simulink model "simulink"  (R2023a)
settings: Solver=VariableStepAuto  StartTime=0.0  StopTime=10.0  RelTol=1e-3
settings Model: Creator=chirag  LastModifiedBy=chirag

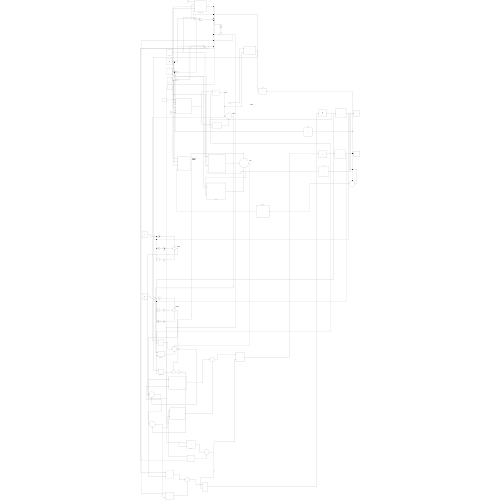
[thumbnail: Simulink's stored preview of the top-level diagram]
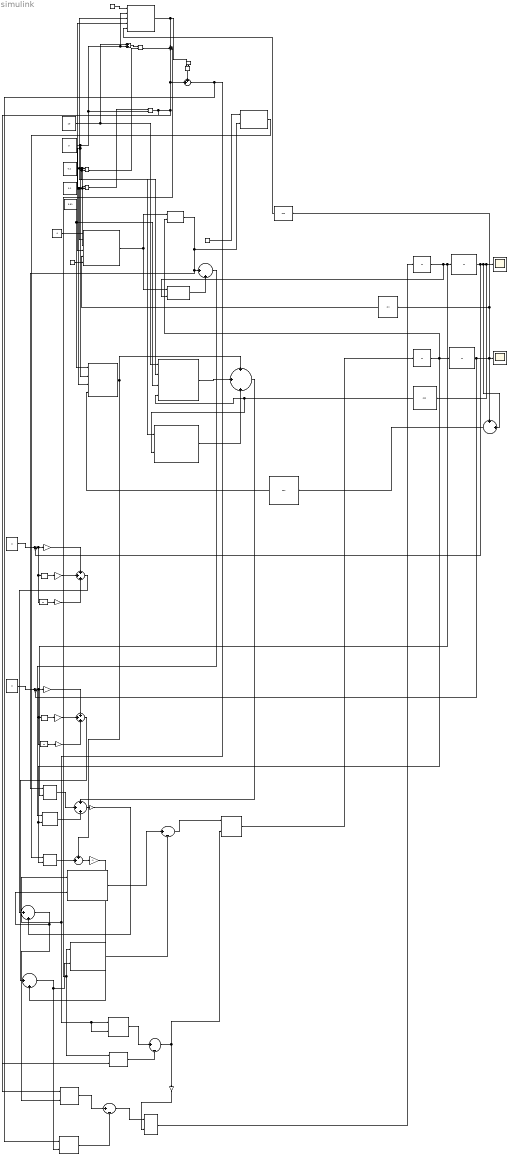
== system simulink ==
  note: G1
  note: tow1
  note: G1
  note: G2
  note: C12
  note: C11
  note: C22
  note: m2
  note: tow2
  (m1+m2)*l^2 : Product
  -m2*l1*l2sin(q2) : Product  Inputs=6
  2*m2*l1*l2*cos(q2) : Product  Inputs=5
  C11*theta1_dot : Product
  C12*thata2_dot : Product
  C22*theta2_dot : Product
  Constant : Constant  Value=2
  Constant1 : Constant  Value=0.5
  Constant2 : Constant  Value=-1
  Constant3 : Constant  Value=-1
  Constant6 : Constant
  Cos(q1) : Trigonometry  Operator=cos
  Cos(q1+q2) : Trigonometry  Operator=cos
  Cos(q2) : Trigonometry  Operator=cos
  Derivative : Derivative
  Derivative1 : Derivative
  Divide : Product  Inputs=*/
  Divide1 : Product  Inputs=*/
  Gain : Gain  Gain=-1
  Gain1 : Gain  Gain=-1
  Gain4 : Gain  Gain=-1
  Integrator : Integrator  InitialCondition=0.1
  Integrator{1,3..5} (4 alike) : Integrator
  Integrator2 : Integrator  InitialCondition=0.1
  KD1 : Gain  Gain=80
  KD2 : Gain  Gain=90
  KI1 : Gain  Gain=80
  KI2 : Gain  Gain=90
  KP1 : Gain  Gain=50
  KP2 : Gain  Gain=60
  M11*M22 : Product
  M12^2 : Product
  Product{,1..3,7,9..11} (8 alike) : Product
  Product4 : Product  Inputs=4
  Sin(q2) : Trigonometry
  Sum : Sum  Inputs=++|
  Sum{1,4,6,8..9} (5 alike) : Sum  Inputs=+++
  Sum10 : Sum  Inputs=++|
  Sum11 : Sum  Inputs=|++
  Sum12 : Sum  Inputs=|++
  Sum{5,7,13..15} (5 alike) : Sum  Inputs=|+-
  Sum2 : Sum  Inputs=|++
  Sum3 : Sum  Inputs=++|
  g : Constant  Value=9.81
  l1 : Constant  Value=0.2
  l1^2 : Product
  l1cos(q1) : Product
  l2 : Constant  Value=0.1
  l2^2 : Product
  m1 : Constant  Value=10
  m1+m2 : Sum
  m1l1gcos(q1) : Product  Inputs=4
  m2 : Constant  Value=5
  m2*l^2 : Product
  q1 : Scope
  q1f : Constant  Value=0
  q2 : Scope
  q2f : Constant  Value=0
  wires:
  Integrator/1 -> Sum5/2, Sum3/2, Cos(q1)/1, q1/1
  Integrator1/1 -> Product3/2, C11*theta1_dot/2, Integrator/1
  Integrator2/1 -> Sum7/2, Sum3/1, q2/1, Cos(q2)/1, Sin(q2)/1
  m1/1 -> m1l1gcos(q1)/1, m1+m2/1
  m2/1 -> Product4/2, -m2*l1*l2sin(q2)/4, m2*l^2/2, 2*m2*l1*l2*cos(q2)/2, m1+m2/2
  m1+m2/1 -> (m1+m2)*l^2/1
  l1^2/1 -> (m1+m2)*l^2/2
  (m1+m2)*l^2/1 -> Sum1/2
  l2^2/1 -> m2*l^2/1
  m2*l^2/1 -> M11*M22/2, Product10/1, Sum1/3, Sum/2
  Constant/1 -> 2*m2*l1*l2*cos(q2)/1
  Cos(q2)/1 -> 2*m2*l1*l2*cos(q2)/5
  2*m2*l1*l2*cos(q2)/1 -> Product/1, Sum1/1
  Product/1 -> Sum/1
  Constant1/1 -> Product/2
  Constant2/1 -> -m2*l1*l2sin(q2)/1
  Sin(q2)/1 -> -m2*l1*l2sin(q2)/5
  Constant3/1 -> Product1/1
  l2/1 -> 2*m2*l1*l2*cos(q2)/4, Product4/3, -m2*l1*l2sin(q2)/2, l2^2/2, l2^2/1
  l1/1 -> m1l1gcos(q1)/2, -m2*l1*l2sin(q2)/3, l1^2/1, l1cos(q1)/1, l1^2/2, 2*m2*l1*l2*cos(q2)/3
  Integrator3/1 -> C22*theta2_dot/2, C12*thata2_dot/2, Product2/2, Integrator2/1
  -m2*l1*l2sin(q2)/1 -> Product2/1, Product3/1
  Product2/1 -> C11*theta1_dot/1, Sum2/1, Product1/2
  Product3/1 -> Sum2/2
  Sum3/1 -> Cos(q1+q2)/1
  g/1 -> m1l1gcos(q1)/3, Product4/1
  Cos(q1+q2)/1 -> Product4/4
  Cos(q1)/1 -> l1cos(q1)/2, m1l1gcos(q1)/4
  Product4/1 -> Sum10/1, Sum4/1
  m1l1gcos(q1)/1 -> Sum4/2
  l1cos(q1)/1 -> Sum4/3
  q1f/1 -> Sum5/1
  Sum5/1 -> Integrator4/1, Derivative/1, KP1/1
  Derivative/1 -> KD1/1
  Integrator4/1 -> KI1/1
  KD1/1 -> Sum6/2
  KP1/1 -> Sum6/1
  KI1/1 -> Sum6/3
  Integrator5/1 -> KI2/1
  KP2/1 -> Sum8/1
  Sum7/1 -> Integrator5/1, Derivative1/1, KP2/1
  KD2/1 -> Sum8/2
  KI2/1 -> Sum8/3
  Derivative1/1 -> KD2/1
  q2f/1 -> Sum7/1
  C11*theta1_dot/1 -> Sum9/2
  Sum2/1 -> C12*thata2_dot/1
  C12*thata2_dot/1 -> Sum9/3
  Sum4/1 -> Sum9/1
  Sum9/1 -> Gain/1
  Product1/1 -> C22*theta2_dot/1
  C22*theta2_dot/1 -> Sum10/2
  Sum10/1 -> Gain1/1
  Sum/1 -> Product11/1, M12^2/2, M12^2/1, Product7/1
  Sum6/1 -> Sum11/1
  Gain/1 -> Sum11/2
  Sum11/1 -> Product10/2, Product7/2
  Sum1/1 -> M11*M22/1, Product9/1
  Sum8/1 -> Sum12/1
  Gain1/1 -> Sum12/2
  Sum12/1 -> Product11/2, Product9/2
  Product7/1 -> Sum13/1
  Product9/1 -> Sum13/2
  M12^2/1 -> Sum14/1
  M11*M22/1 -> Sum14/2
  Sum13/1 -> Divide/1
  Sum14/1 -> Divide/2, Gain4/1
  Divide/1 -> Integrator3/1
  Product10/1 -> Sum15/1
  Product11/1 -> Sum15/2
  Sum15/1 -> Divide1/1
  Gain4/1 -> Divide1/2
  Divide1/1 -> Integrator1/1
  Constant6/1 -> -m2*l1*l2sin(q2)/6
